simulink model "Opportunity_Finder"  (R2019b)
settings: Solver=ode1  StartTime=0.0  StopTime=Inf  FixedStep=0.001  RelTol=1e-3
PostLoadFcn:
  | , if any(exist('dsrtsu_mdlpostloadfcn', 'file') == [2, 3, 6]), try dsrtsu_mdlpostloadfcn('Execute', bdroot); catch fprintf('Error in PostLoadFcn (dsrtsu_mdlpostloadfcn) for model "%s":\n %s\n', bdroot, lasterr); end, end,
Description:
  | Standard RTI1401 template.
  | Supported MATLAB version:  R2018b.
settings Model: Tag=RTI1401  DSRTSU_INTERNAL_RTI_VER=540  DSRTSU_INTERNAL_RTI_TYPE=rti1401  RTICANMMDATA=struct('GeneralSetupData',struct('modelroot','C:\Users\linqi\Desktop\matlab\ACC\CarMaker','generalsettings',struct('filesettings',struct('destfolder',struct('Name','RTICANMM_FILES','Check',1),'buildfolder',struct('Name','.','Check',1),'AbsDestfolder',struct('Name','C:\Users\linqi\Desktop\matlab\ACC\CarMaker\RTICANMM_FILES'),'AbsBuildfolder',struct('Name','C:\Users\linqi\Desktop\matlab\ACC\CarMaker'))),'options',struct('addpaths',1,'rmpaths',1,'addtrcexclusion',logical(1),'cannavigator',struct('checkmonitoring',0),'show_usrtrc',0,'use_usrtrc',0),'advanced',struct('options',ones(1,100)),'MPSetup',{{}},'RTI',struct('Type','RTI1401','Ver','7.12','Date','02-May-2019'),'modelname','Opportunity_Finder','block','Opportunity_Finder'))  DSRTSU_INTERNAL_RTIFPGA=130  Creator=linqi  LastModifiedBy=lenovo
settings DataIOCC: ReturnWorkspaceOutputs=off
settings OptimizationCC: BlockReduction=off  OptimizeBlockIOStorage=off  BufferReuse=off  GlobalBufferReuse=off  ExpressionFolding=off  LocalBlockOutputs=off  OptimizeDataStoreBuffers=off  BusAssignmentInplaceUpdate=off
settings DebuggingCC: ArithmeticOperatorsInVariantConditions=warning
settings HardwareCC: ProdBitPerPointer=32  ProdBitPerSizeT=32  ProdBitPerPtrDiffT=32  ProdLargestAtomicInteger=Integer  ProdEndianess=BigEndian  ProdWordSize=32  ProdHWDeviceType=Custom Processor->Custom  TargetIntDivRoundTo=Zero  TargetEndianess=BigEndian  TargetHWDeviceType=Custom Processor->Custom
settings SFSimCC: SimUseLocalCustomCode=off  MATLABDynamicMemAlloc=off  CustomCodeUndefinedFunction=UseInterfaceOnly
settings RTWCC: Description=dSPACE DS1401 Hardware Platform  SystemTargetFile=rti1401.tlc  MakeCommand=make_rti  TemplateMakefile=rti1401.tmf  RTWUseLocalCustomCode=off
settings CodeAppCC: StateflowObjectComments=on
settings STFCustomTargetCC: ParMdlRefBuildCompliant=on  MatFileLogging=on  SystemTargetFile=rti1401.tlc
settings GRTTargetCC: TargetLangStandard=C89/C90 (ANSI)  CompOptLevelCompliant=off  ConcurrentExecutionCompliant=off  CombineOutputUpdateFcns=off  CPPClassGenCompliant=off  UseToolchainInfoCompliant=off
settings ConfigComp: CovMetricSettings=dswe

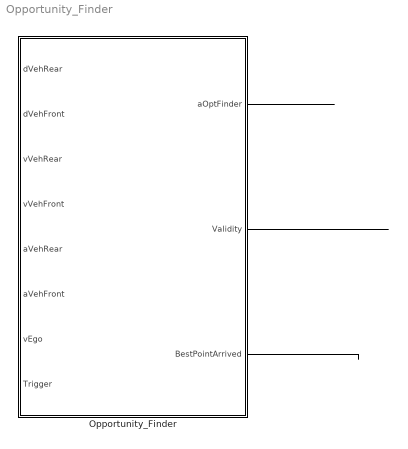
== system Opportunity_Finder ==
  Opportunity_Finder : MATLAB Function  TreatAsAtomicUnit=on
  wires:
  Opportunity_Finder/2(Validity) -> ?
  Opportunity_Finder/3(BestPointArrived) -> ?
  Opportunity_Finder/1(aOptFinder) -> ?

== matlab function Opportunity_Finder/Opportunity_Finder ==
  data: dVehRear input; dVehFront input; aOptFinder output; vVehRear input; vVehFront input; aVehRear input; aVehFront input; vEgo input; Trigger input; Validity output; BestPointArrived output
function [aOptFinder,Validity,BestPointArrived] = Opportunity_Finder(dVehRear,dVehFront,vVehRear,vVehFront,aVehRear,aVehFront,vEgo,Trigger)
if Trigger == 1
    dt = 0.1;
    dVehInit = [dVehRear dVehFront]; %[dRear,dFront]
    vVehInit = [30 vVehFront]; %[vRear,vFront] m/s
    aVehInit = [aVehRear aVehFront]; %[aRear,aFront]
    vEgoInit = vEgo;
    T = 8/2.3;
    w = [4;1;1;1];
    i = 1;
    CDistance = zeros(315,1);
    CTTCRear = zeros(315,1);
    CTTCFront = zeros(315,1);
    CTTC = zeros(315,1);
    CAccel = zeros(315,1);
    CTime = zeros(315,1);
    CAdjust = zeros(315,1);
    aResult = zeros(315,1);
    tResult = zeros(315,1);
    for a = -1:0.1:1
        for t = 1:0.5:8        
            dVeh = dVehInit + (vVehInit+aVehInit*t)*t + aVehInit*(t^2)*exp(-t/T) - aVehInit*t^2;
            vVeh = -T*aVehInit*exp(-t/T) + vVehInit + aVehInit*t;
            dEgo = vEgoInit*t + 0.5*a*t^2;
            vEgo = vEgoInit + a*t;
            CDistance(i) = calcCostDistance(dVeh(1),dVeh(2),dEgo);
            CTTCRear(i) = calcCTTC(dVeh(1),vVeh(1),dEgo,vEgo);
            CTTCFront(i) = calcCTTC(dVeh(2),vVeh(2),dEgo,vEgo);
            CTTC(i) = 0.5*(CTTCRear(i)+CTTCFront(i));
            CAccel(i) = calcCAccel(a);
            CTime(i) = calcCTime(t);
            CAdjust(i) = [CDistance(i) CTTC(i) CAccel(i) CTime(i)]*w; 
            aResult(i) = a;
            tResult(i) = t;
            i = i+1;
        end
    end
    [cMin,iMin] = min(CAdjust);
    aOptFinder = aResult(iMin);
    Validity = 1;
else
    aOptFinder = 0;
    Validity = 0;
end
CurrentCDistance = calcCostDistance(dVehInit(1),dVehInit(2),0);
if CurrentCDistance < 0.1
    BestPointArrived = 1;
else
    BestPointArrived = 0;
end

end


function [CDistance] = calcCostDistance(dVehRear,dVehFront,dEgo)
dPercentage = (dEgo-dVehRear)/(dVehFront-dVehRear);
dPercentage = max(min(dPercentage,1),0);
CDistance = interp1([0 0.4 0.6 1],[1 0 0 1],dPercentage,'linear');
end

function [CAccel] = calcCAccel(a)
CAccel = interp1([0 1 2],[0 0.4 1],abs(a),'linear');
end

function [CTime] = calcCTime(t)
CTime = interp1([0 8],[0 1],t,'linear');
end

function [CTTC] = calcCTTC(dVeh,vVeh,dEgo,vEgo)

vDiff = vVeh - vEgo;
dDiff = dVeh - dEgo;

if abs(vDiff)<0.1
    TTC = 255;
elseif sign(dDiff) == sign(vDiff)
    TTC = 255;
else
    TTC = abs(dDiff/vDiff);
end
TTC = min(max(TTC,0),5);
CTTC = interp1([0 3 5],[1 0 0],TTC,'linear');
    
end
